simulink model "InPark_Test"  (R2025b)
settings: Solver=VariableStepAuto  StartTime=0.0  StopTime=10.0  RelTol=1e-3
libraries: MyPMSMLibrary x1
settings Model: Creator=jff_1  LastModifiedBy=jff_1

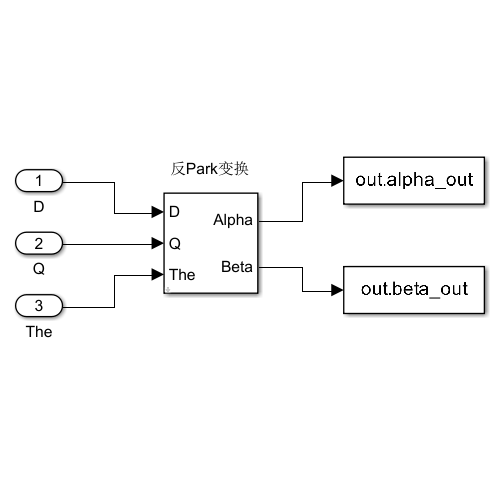
[thumbnail: Simulink's stored preview of the top-level diagram]
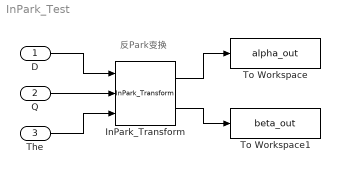
== system InPark_Test ==
  note: 反Park变换
  D : Inport
  Q : Inport  Port=2
  The : Inport  Port=3
  InPark_Transform : MyPMSMLibrary/Transforms/InPark_Transform
  To Workspace : ToWorkspace  VariableName=alpha_out  SampleTime=-1
  To Workspace1 : ToWorkspace  VariableName=beta_out  SampleTime=-1
  wires:
  D/1 -> InPark_Transform/1
  Q/1 -> InPark_Transform/2
  The/1 -> InPark_Transform/3
  InPark_Transform/1 -> To Workspace/1
  InPark_Transform/2 -> To Workspace1/1
